simulink model "AoAIOLoopSystem"  (R2020a)
settings: Solver=VariableStepAuto  StartTime=0.0  StopTime=10.0  RelTol=1e-3
settings Model: Creator=OZAN  LastModifiedBy=OZAN

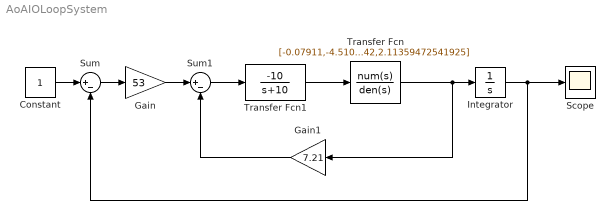
== system AoAIOLoopSystem ==
  Constant : Constant
  Gain : Gain  Gain=53
  Gain1 : Gain  Gain=7.21
  Integrator : Integrator
  Scope : Scope
  Sum : Sum  Inputs=|+-
  Sum1 : Sum  Inputs=|+-
  Transfer Fcn : TransferFcn  Numerator=[-0.07911,-4.51081350665340,0]  Denominator=[1,0.872456756315742,2.11359472541925]
  Transfer Fcn1 : TransferFcn  Numerator=[-10]  Denominator=[1 10]
  wires:
  Constant/1 -> Sum/1
  Transfer Fcn1/1 -> Transfer Fcn/1
  Sum1/1 -> Transfer Fcn1/1
  Sum/1 -> Gain/1
  Gain/1 -> Sum1/1
  Integrator/1 -> Scope/1, Sum/2
  Gain1/1 -> Sum1/2
  Transfer Fcn/1 -> Gain1/1, Integrator/1
